simulink model "prepFixedPointControl"  (R2023a)
settings: Solver=VariableStepAuto  StartTime=0.0  StopTime=10.0  RelTol=1e-3
libraries: mci_models x2
settings Model: Creator=fluky  LastModifiedBy=fluky

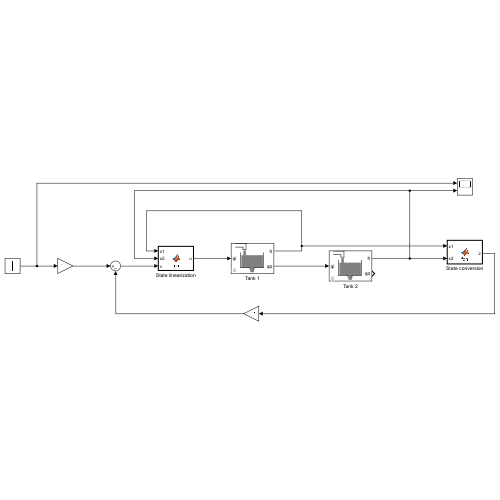
[thumbnail: Simulink's stored preview of the top-level diagram]
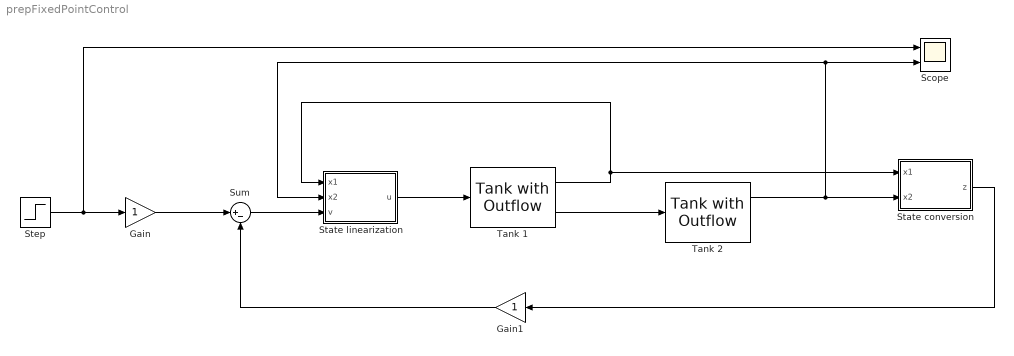
== system prepFixedPointControl ==
  Gain : Gain
  Gain1 : Gain
  Scope : Scope  NumInputPorts=2
  State conversion : MATLAB Function  TreatAsAtomicUnit=on
  State linearization : MATLAB Function  TreatAsAtomicUnit=on
  Step : Step  SampleTime=0
  Sum : Sum  Inputs=|+-
  Tank 1 : mci_models/Fluid Systems/Tank with Outflow  At=0.00528101  Ao=0.0005309  rho=1000  zeta=0.05  g=9.81  h0=0
  Tank 2 : mci_models/Fluid Systems/Tank with Outflow  At=0.00528101  Ao=0.0005309  rho=1000  zeta=0.05  g=9.81  h0=0
  wires:
  Tank 1/2 -> Tank 2/1
  State linearization/1(u) -> Tank 1/1
  Sum/1 -> State linearization/3(v)
  Gain/1 -> Sum/1
  Gain1/1 -> Sum/2
  State conversion/1(z) -> Gain1/1
  Tank 2/1 -> State conversion/2(x2), State linearization/2(x2), Scope/2
  Tank 1/1 -> State linearization/1(x1), State conversion/1(x1)
  Step/1 -> Scope/1, Gain/1

== matlab function prepFixedPointControl/State linearization ==
  data: x1 input; u output; x2 input; v input
function u = fcn(x1, x2, v)

y = x1 * x2 * v;

== matlab function prepFixedPointControl/State conversion ==
  data: x1 input; z output; x2 input
function z = fcn(x1, x2)

y = x1 * x2;
